simulink model "w3_warplab_trigger_proc"  (Simulink 7.7)
settings: Solver=ode45  StartTime=0.0  StopTime=100  RelTol=1e-3
InitFcn:
  | warplab_trigger_proc_init
StartFcn:
  | warplab_trigger_proc_init
undefined symbols (not defined in the file or in its folder): gcbh, xlBlockLoadCallback, xlGetNormalizedPeriod
libraries: xbsIndex_r4 x817, xbsEDKLib_r4 x1
(part 3 of 6)

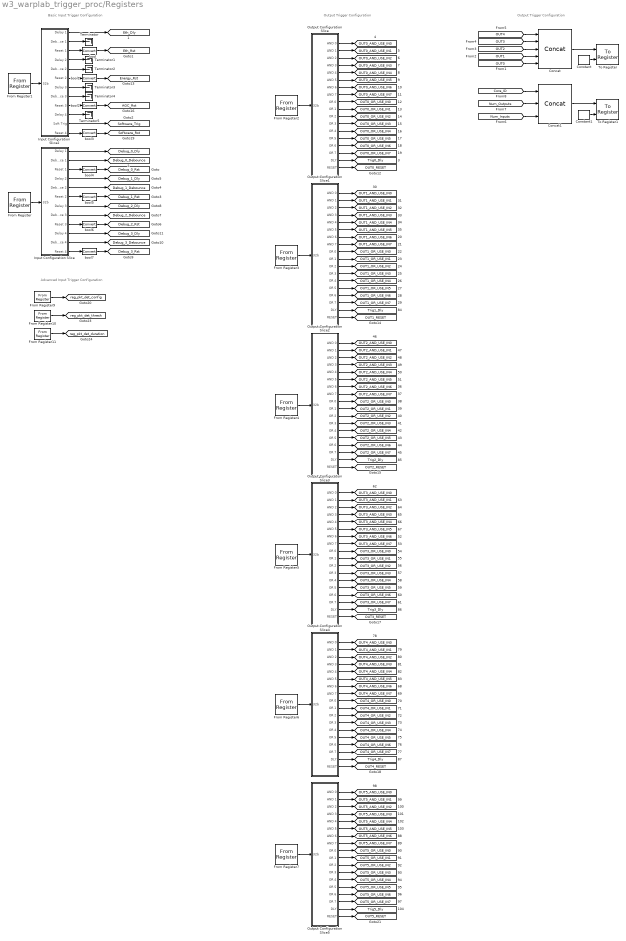
== system w3_warplab_trigger_proc/Registers ==
  note: Basic Input Trigger Configuration
  note: Advanced Input Trigger Configuration
  note: Output Trigger Configuration
  note: Output Trigger Configuration
  Concat : xbsIndex_r4/Concat  num_inputs=5  dbl_ovrd=off  block_type=concat
  Concat1 : xbsIndex_r4/Concat  num_inputs=3  dbl_ovrd=off  block_type=concat
  Constant : xbsIndex_r4/Constant  const=1  gui_display_data_type=Boolean  arith_type=Boolean  n_bits=16  bin_pt=14  preci_type=Single  exp_width=8  frac_width=24  explicit_period=off  period=1  equ=P=C  opselect=C  inp2=PCIN>>17  opr=+  inp1=P  carry=CIN  dbl_ovrd=off  block_type=constant
  Constant1 : xbsIndex_r4/Constant  const=1  gui_display_data_type=Boolean  arith_type=Boolean  n_bits=16  bin_pt=14  preci_type=Single  exp_width=8  frac_width=24  explicit_period=off  period=1  equ=P=C  opselect=C  inp2=PCIN>>17  opr=+  inp1=P  carry=CIN  dbl_ovrd=off  block_type=constant
  From Register : xbsIndex_r4/From Register  shared_memory_name='TRIG_CONF_INBANK1'  init=IN_BANK1  period=1  ownership=Locally owned and initialized  gui_display_data_type=Fixed-point  arith_type=Unsigned  n_bits=32  bin_pt=0  preci_type=Single  dbl_ovrd=off  block_type=fromreg
      settings: AttributesFormatString=<< %<shared_memory_name> >>  infoedit="Register block that reads data to a shared memory register.  Delay of one sample period."
  From Register1 : xbsIndex_r4/From Register  shared_memory_name='TRIG_CONF_INBANK0'  init=IN_BANK0  period=1  ownership=Locally owned and initialized  gui_display_data_type=Fixed-point  arith_type=Unsigned  n_bits=32  bin_pt=0  preci_type=Single  dbl_ovrd=off  block_type=fromreg
      settings: AttributesFormatString=<< %<shared_memory_name> >>  infoedit="Register block that reads data to a shared memory register.  Delay of one sample period."
  From Register10 : xbsIndex_r4/From Register  shared_memory_name='RSSI_PKT_DET_THRESHOLDS'  init=0  period=1  ownership=Locally owned and initialized  gui_display_data_type=Fixed-point  arith_type=Unsigned  n_bits=32  bin_pt=0  preci_type=Single  dbl_ovrd=off  block_type=fromreg
      settings: AttributesFormatString=<< %<shared_memory_name> >>  infoedit="Register block that reads data to a shared memory register.  Delay of one sample period."  block_version=8.2
  From Register11 : xbsIndex_r4/From Register  shared_memory_name='RSSI_PKT_DET_DURATIONS'  init=0  period=1  ownership=Locally owned and initialized  gui_display_data_type=Fixed-point  arith_type=Unsigned  n_bits=32  bin_pt=0  preci_type=Single  dbl_ovrd=off  block_type=fromreg
      settings: AttributesFormatString=<< %<shared_memory_name> >>  infoedit="Register block that reads data to a shared memory register.  Delay of one sample period."  block_version=8.2
  From Register2 : xbsIndex_r4/From Register  shared_memory_name='TRIG_CONF_OUT0'  init=OUT0  period=1  ownership=Locally owned and initialized  gui_display_data_type=Fixed-point  arith_type=Unsigned  n_bits=32  bin_pt=0  preci_type=Single  dbl_ovrd=off  block_type=fromreg
      settings: AttributesFormatString=<< %<shared_memory_name> >>  infoedit="Register block that reads data to a shared memory register.  Delay of one sample period."
  From Register3 : xbsIndex_r4/From Register  shared_memory_name='TRIG_CONF_OUT1'  init=OUT1  period=1  ownership=Locally owned and initialized  gui_display_data_type=Fixed-point  arith_type=Unsigned  n_bits=32  bin_pt=0  preci_type=Single  dbl_ovrd=off  block_type=fromreg
      settings: AttributesFormatString=<< %<shared_memory_name> >>  infoedit="Register block that reads data to a shared memory register.  Delay of one sample period."
  From Register4 : xbsIndex_r4/From Register  shared_memory_name='TRIG_CONF_OUT2'  init=OUT2  period=1  ownership=Locally owned and initialized  gui_display_data_type=Fixed-point  arith_type=Unsigned  n_bits=32  bin_pt=0  preci_type=Single  dbl_ovrd=off  block_type=fromreg
      settings: AttributesFormatString=<< %<shared_memory_name> >>  infoedit="Register block that reads data to a shared memory register.  Delay of one sample period."
  From Register5 : xbsIndex_r4/From Register  shared_memory_name='TRIG_CONF_OUT3'  init=OUT3  period=1  ownership=Locally owned and initialized  gui_display_data_type=Fixed-point  arith_type=Unsigned  n_bits=32  bin_pt=0  preci_type=Single  dbl_ovrd=off  block_type=fromreg
      settings: AttributesFormatString=<< %<shared_memory_name> >>  infoedit="Register block that reads data to a shared memory register.  Delay of one sample period."
  From Register6 : xbsIndex_r4/From Register  shared_memory_name='TRIG_CONF_OUT4'  init=OUT4  period=1  ownership=Locally owned and initialized  gui_display_data_type=Fixed-point  arith_type=Unsigned  n_bits=32  bin_pt=0  preci_type=Single  dbl_ovrd=off  block_type=fromreg
      settings: AttributesFormatString=<< %<shared_memory_name> >>  infoedit="Register block that reads data to a shared memory register.  Delay of one sample period."
  From Register7 : xbsIndex_r4/From Register  shared_memory_name='TRIG_CONF_OUT5'  init=OUT5  period=1  ownership=Locally owned and initialized  gui_display_data_type=Fixed-point  arith_type=Unsigned  n_bits=32  bin_pt=0  preci_type=Single  dbl_ovrd=off  block_type=fromreg
      settings: AttributesFormatString=<< %<shared_memory_name> >>  infoedit="Register block that reads data to a shared memory register.  Delay of one sample period."
  From Register9 : xbsIndex_r4/From Register  shared_memory_name='RSSI_PKT_DET_CONFIG'  init=0  period=1  ownership=Locally owned and initialized  gui_display_data_type=Fixed-point  arith_type=Unsigned  n_bits=32  bin_pt=0  preci_type=Single  dbl_ovrd=off  block_type=fromreg
      settings: AttributesFormatString=<< %<shared_memory_name> >>  infoedit="Register block that reads data to a shared memory register.  Delay of one sample period."  block_version=8.2
  Input Configuration Slice : Subsystem
  Input Configuration Slice2 : Subsystem
  Output Configuration Slice : Subsystem
  Output Configuration Slice1 : Subsystem
  Output Configuration Slice2 : Subsystem
  Output Configuration Slice3 : Subsystem
  Output Configuration Slice4 : Subsystem
  Output Configuration Slice5 : Subsystem
  Terminator{,1..5} (6 alike) : Terminator
  To Register : xbsIndex_r4/To Register  shared_memory_name='TRIG_OUT'  init=0  ownership=Locally owned and initialized  explicit_data_type=on  gui_display_data_type=Fixed-point  arith_type=Unsigned  n_bits=5  bin_pt=0  preci_type=Single  dbl_ovrd=off  block_type=toreg
      settings: AttributesFormatString=<< %<shared_memory_name> >>  infoedit="Register block that writes data to a shared memory register.  Delay of one sample period."
  To Register1 : xbsIndex_r4/To Register  shared_memory_name='CORE_INFO'  init=0  ownership=Locally owned and initialized  explicit_data_type=on  gui_display_data_type=Fixed-point  arith_type=Unsigned  n_bits=24  bin_pt=0  preci_type=Single  dbl_ovrd=off  block_type=toreg
      settings: AttributesFormatString=<< %<shared_memory_name> >>  infoedit="Register block that writes data to a shared memory register.  Delay of one sample period."
  bool{,1..7} (8 alike) : xbsIndex_r4/Convert  gui_display_data_type=Boolean  arith_type=Boolean  n_bits=16  bin_pt=14  float_type=Single  exp_bits=8  fraction_bits=24  quantization=Truncate  overflow=Wrap  en=off  latency=0  dbl_ovrd=off  pipeline=off  block_type=convert
  tag scope: AGC_Rst=global, Debug_0_Debounce=global, Debug_0_Dly=global, Debug_0_Rst=global, Debug_1_Debounce=global, Debug_1_Dly=global, Debug_1_Rst=global, Debug_2_Debounce=global, Debug_2_Dly=global, Debug_2_Rst=global, Debug_3_Debounce=global, Debug_3_Dly=global, Debug_3_Rst=global, Energy_Rst=global, Eth_Dly=global, Eth_Rst=global, OUT0_AND_USE_IN0=global, OUT0_AND_USE_IN1=global, OUT0_AND_USE_IN2=global, OUT0_AND_USE_IN3=global, OUT0_AND_USE_IN4=global, OUT0_AND_USE_IN5=global, OUT0_AND_USE_IN6=global, OUT0_AND_USE_IN7=global, OUT0_OR_USE_IN0=global, OUT0_OR_USE_IN1=global, OUT0_OR_USE_IN2=global, OUT0_OR_USE_IN3=global, OUT0_OR_USE_IN4=global, OUT0_OR_USE_IN5=global, OUT0_OR_USE_IN6=global, OUT0_OR_USE_IN7=global, OUT0_RESET=global, OUT1_AND_USE_IN0=global, OUT1_AND_USE_IN1=global, OUT1_AND_USE_IN2=global, OUT1_AND_USE_IN3=global, OUT1_AND_USE_IN4=global, OUT1_AND_USE_IN5=global, OUT1_AND_USE_IN6=global, OUT1_AND_USE_IN7=global, OUT1_OR_USE_IN0=global, OUT1_OR_USE_IN1=global, OUT1_OR_USE_IN2=global, OUT1_OR_USE_IN3=global, OUT1_OR_USE_IN4=global, OUT1_OR_USE_IN5=global, OUT1_OR_USE_IN6=global, OUT1_OR_USE_IN7=global, OUT1_RESET=global, OUT2_AND_USE_IN0=global, OUT2_AND_USE_IN1=global, OUT2_AND_USE_IN2=global, OUT2_AND_USE_IN3=global, OUT2_AND_USE_IN4=global, OUT2_AND_USE_IN5=global, OUT2_AND_USE_IN6=global, OUT2_AND_USE_IN7=global, OUT2_OR_USE_IN0=global, OUT2_OR_USE_IN1=global, OUT2_OR_USE_IN2=global, OUT2_OR_USE_IN3=global, OUT2_OR_USE_IN4=global, OUT2_OR_USE_IN5=global, OUT2_OR_USE_IN6=global, OUT2_OR_USE_IN7=global, OUT2_RESET=global, OUT3_AND_USE_IN0=global, OUT3_AND_USE_IN1=global, OUT3_AND_USE_IN2=global, OUT3_AND_USE_IN3=global, OUT3_AND_USE_IN4=global, OUT3_AND_USE_IN5=global, OUT3_AND_USE_IN6=global, OUT3_AND_USE_IN7=global, OUT3_OR_USE_IN0=global, OUT3_OR_USE_IN1=global, OUT3_OR_USE_IN2=global, OUT3_OR_USE_IN3=global, OUT3_OR_USE_IN4=global, OUT3_OR_USE_IN5=global, OUT3_OR_USE_IN6=global, OUT3_OR_USE_IN7=global, OUT3_RESET=global, OUT4_AND_USE_IN0=global, OUT4_AND_USE_IN1=global, OUT4_AND_USE_IN2=global, OUT4_AND_USE_IN3=global, OUT4_AND_USE_IN4=global, OUT4_AND_USE_IN5=global, OUT4_AND_USE_IN6=global, OUT4_AND_USE_IN7=global, OUT4_OR_USE_IN0=global, OUT4_OR_USE_IN1=global, OUT4_OR_USE_IN2=global, OUT4_OR_USE_IN3=global, OUT4_OR_USE_IN4=global, OUT4_OR_USE_IN5=global, OUT4_OR_USE_IN6=global, OUT4_OR_USE_IN7=global, OUT4_RESET=global, OUT5_AND_USE_IN0=global, OUT5_AND_USE_IN1=global, OUT5_AND_USE_IN2=global, OUT5_AND_USE_IN3=global, OUT5_AND_USE_IN4=global, OUT5_AND_USE_IN5=global, OUT5_AND_USE_IN6=global, OUT5_AND_USE_IN7=global, OUT5_OR_USE_IN0=global, OUT5_OR_USE_IN1=global, OUT5_OR_USE_IN2=global, OUT5_OR_USE_IN3=global, OUT5_OR_USE_IN4=global, OUT5_OR_USE_IN5=global, OUT5_OR_USE_IN6=global, OUT5_OR_USE_IN7=global, OUT5_RESET=global, Software_Rst=global, Software_Trig=global, Trig0_Dly=global, Trig1_Dly=global, Trig2_Dly=global, Trig3_Dly=global, Trig4_Dly=global, Trig5_Dly=global, reg_pkt_det_config=global, reg_pkt_det_duration=global, reg_pkt_det_thresh=global
  wires:
  Input Configuration Slice/1(Delay 1) -> [Debug_0_Dly]
  Input Configuration Slice/2(Debounce 1) -> [Debug_0_Debounce]
  Input Configuration Slice/3(Reset 1) -> bool4/1
  Input Configuration Slice/4(Delay 2) -> [Debug_1_Dly]
  Input Configuration Slice/5(Debounce 2) -> [Debug_1_Debounce]
  Input Configuration Slice/6(Reset 2) -> bool5/1
  Input Configuration Slice/7(Delay 3) -> [Debug_2_Dly]
  Input Configuration Slice/8(Debounce 3) -> [Debug_2_Debounce]
  Input Configuration Slice/9(Reset 3) -> bool6/1
  Input Configuration Slice/10(Delay 4) -> [Debug_3_Dly]
  Input Configuration Slice/11(Debounce 4) -> [Debug_3_Debounce]
  Input Configuration Slice/12(Reset 4) -> bool7/1
  From Register/1 -> Input Configuration Slice/1(32b)
  Input Configuration Slice2/1(Delay 1) -> [Eth_Dly]
  Input Configuration Slice2/2(Debounce 1) -> Terminator/1
  Input Configuration Slice2/3(Reset 1) -> bool/1
  Input Configuration Slice2/4(Delay 2) -> Terminator1/1
  Input Configuration Slice2/5(Debounce 2) -> Terminator2/1
  Input Configuration Slice2/6(Reset 2) -> bool1/1
  Input Configuration Slice2/7(Delay 3) -> Terminator3/1
  Input Configuration Slice2/8(Debounce 3) -> Terminator4/1
  Input Configuration Slice2/9(Reset 3) -> bool2/1
  Input Configuration Slice2/10(Delay 4) -> Terminator5/1
  Input Configuration Slice2/11(Soft Trig) -> [Software_Trig]
  Input Configuration Slice2/12(Reset 4) -> bool3/1
  From Register1/1 -> Input Configuration Slice2/1(32b)
  From Register9/1 -> [reg_pkt_det_config]
  From Register10/1 -> [reg_pkt_det_thresh]
  From Register11/1 -> [reg_pkt_det_duration]
  From Register2/1 -> Output Configuration Slice/1(32b)
  Output Configuration Slice/1(AND 0) -> [OUT0_AND_USE_IN0]
  Output Configuration Slice/2(AND 1) -> [OUT0_AND_USE_IN1]
  Output Configuration Slice/3(AND 2) -> [OUT0_AND_USE_IN2]
  Output Configuration Slice/4(AND 3) -> [OUT0_AND_USE_IN3]
  Output Configuration Slice/5(AND 4) -> [OUT0_AND_USE_IN4]
  Output Configuration Slice/6(AND 5) -> [OUT0_AND_USE_IN5]
  Output Configuration Slice/7(AND 6) -> [OUT0_AND_USE_IN6]
  Output Configuration Slice/8(AND 7) -> [OUT0_AND_USE_IN7]
  Output Configuration Slice/9(OR 0) -> [OUT0_OR_USE_IN0]
  Output Configuration Slice/10(OR 1) -> [OUT0_OR_USE_IN1]
  Output Configuration Slice/11(OR 2) -> [OUT0_OR_USE_IN2]
  Output Configuration Slice/12(OR 3) -> [OUT0_OR_USE_IN3]
  Output Configuration Slice/13(OR 4) -> [OUT0_OR_USE_IN4]
  Output Configuration Slice/14(OR 5) -> [OUT0_OR_USE_IN5]
  Output Configuration Slice/15(OR 6) -> [OUT0_OR_USE_IN6]
  Output Configuration Slice/16(OR 7) -> [OUT0_OR_USE_IN7]
  Output Configuration Slice/18(RESET) -> [OUT0_RESET]
  Output Configuration Slice1/1(AND 0) -> [OUT1_AND_USE_IN0]
  Output Configuration Slice1/2(AND 1) -> [OUT1_AND_USE_IN1]
  Output Configuration Slice1/3(AND 2) -> [OUT1_AND_USE_IN2]
  Output Configuration Slice1/4(AND 3) -> [OUT1_AND_USE_IN3]
  Output Configuration Slice1/5(AND 4) -> [OUT1_AND_USE_IN4]
  Output Configuration Slice1/6(AND 5) -> [OUT1_AND_USE_IN5]
  Output Configuration Slice1/7(AND 6) -> [OUT1_AND_USE_IN6]
  Output Configuration Slice1/8(AND 7) -> [OUT1_AND_USE_IN7]
  Output Configuration Slice1/9(OR 0) -> [OUT1_OR_USE_IN0]
  Output Configuration Slice1/10(OR 1) -> [OUT1_OR_USE_IN1]
  Output Configuration Slice1/11(OR 2) -> [OUT1_OR_USE_IN2]
  Output Configuration Slice1/12(OR 3) -> [OUT1_OR_USE_IN3]
  Output Configuration Slice1/13(OR 4) -> [OUT1_OR_USE_IN4]
  Output Configuration Slice1/14(OR 5) -> [OUT1_OR_USE_IN5]
  Output Configuration Slice1/15(OR 6) -> [OUT1_OR_USE_IN6]
  Output Configuration Slice1/16(OR 7) -> [OUT1_OR_USE_IN7]
  Output Configuration Slice2/1(AND 0) -> [OUT2_AND_USE_IN0]
  Output Configuration Slice2/2(AND 1) -> [OUT2_AND_USE_IN1]
  Output Configuration Slice2/3(AND 2) -> [OUT2_AND_USE_IN2]
  Output Configuration Slice2/4(AND 3) -> [OUT2_AND_USE_IN3]
  Output Configuration Slice2/5(AND 4) -> [OUT2_AND_USE_IN4]
  Output Configuration Slice2/6(AND 5) -> [OUT2_AND_USE_IN5]
  Output Configuration Slice2/7(AND 6) -> [OUT2_AND_USE_IN6]
  Output Configuration Slice2/8(AND 7) -> [OUT2_AND_USE_IN7]
  Output Configuration Slice2/9(OR 0) -> [OUT2_OR_USE_IN0]
  Output Configuration Slice2/10(OR 1) -> [OUT2_OR_USE_IN1]
  Output Configuration Slice2/11(OR 2) -> [OUT2_OR_USE_IN2]
  Output Configuration Slice2/12(OR 3) -> [OUT2_OR_USE_IN3]
  Output Configuration Slice2/13(OR 4) -> [OUT2_OR_USE_IN4]
  Output Configuration Slice2/14(OR 5) -> [OUT2_OR_USE_IN5]
  Output Configuration Slice2/15(OR 6) -> [OUT2_OR_USE_IN6]
  Output Configuration Slice2/16(OR 7) -> [OUT2_OR_USE_IN7]
  Output Configuration Slice3/1(AND 0) -> [OUT3_AND_USE_IN0]
  Output Configuration Slice3/2(AND 1) -> [OUT3_AND_USE_IN1]
  Output Configuration Slice3/3(AND 2) -> [OUT3_AND_USE_IN2]
  Output Configuration Slice3/4(AND 3) -> [OUT3_AND_USE_IN3]
  Output Configuration Slice3/5(AND 4) -> [OUT3_AND_USE_IN4]
  Output Configuration Slice3/6(AND 5) -> [OUT3_AND_USE_IN5]
  Output Configuration Slice3/7(AND 6) -> [OUT3_AND_USE_IN6]
  Output Configuration Slice3/8(AND 7) -> [OUT3_AND_USE_IN7]
  Output Configuration Slice3/9(OR 0) -> [OUT3_OR_USE_IN0]
  Output Configuration Slice3/10(OR 1) -> [OUT3_OR_USE_IN1]
  Output Configuration Slice3/11(OR 2) -> [OUT3_OR_USE_IN2]
  Output Configuration Slice3/12(OR 3) -> [OUT3_OR_USE_IN3]
  Output Configuration Slice3/13(OR 4) -> [OUT3_OR_USE_IN4]
  Output Configuration Slice3/14(OR 5) -> [OUT3_OR_USE_IN5]
  Output Configuration Slice3/15(OR 6) -> [OUT3_OR_USE_IN6]
  Output Configuration Slice3/16(OR 7) -> [OUT3_OR_USE_IN7]
  Output Configuration Slice4/1(AND 0) -> [OUT4_AND_USE_IN0]
  Output Configuration Slice4/2(AND 1) -> [OUT4_AND_USE_IN1]
  Output Configuration Slice4/3(AND 2) -> [OUT4_AND_USE_IN2]
  Output Configuration Slice4/4(AND 3) -> [OUT4_AND_USE_IN3]
  Output Configuration Slice4/5(AND 4) -> [OUT4_AND_USE_IN4]
  Output Configuration Slice4/6(AND 5) -> [OUT4_AND_USE_IN5]
  Output Configuration Slice4/7(AND 6) -> [OUT4_AND_USE_IN6]
  Output Configuration Slice4/8(AND 7) -> [OUT4_AND_USE_IN7]
  Output Configuration Slice4/9(OR 0) -> [OUT4_OR_USE_IN0]
  Output Configuration Slice4/10(OR 1) -> [OUT4_OR_USE_IN1]
  Output Configuration Slice4/11(OR 2) -> [OUT4_OR_USE_IN2]
  Output Configuration Slice4/12(OR 3) -> [OUT4_OR_USE_IN3]
  Output Configuration Slice4/13(OR 4) -> [OUT4_OR_USE_IN4]
  Output Configuration Slice4/14(OR 5) -> [OUT4_OR_USE_IN5]
  Output Configuration Slice4/15(OR 6) -> [OUT4_OR_USE_IN6]
  Output Configuration Slice4/16(OR 7) -> [OUT4_OR_USE_IN7]
  [OUT4] -> Concat/1
  [OUT3] -> Concat/2
  [OUT2] -> Concat/3
  [OUT1] -> Concat/4
  [OUT0] -> Concat/5
  Concat/1 -> To Register/1
  Constant/1 -> To Register/2
  bool/1 -> [Eth_Rst]
  bool1/1 -> [Energy_Rst]
  bool2/1 -> [AGC_Rst]
  bool3/1 -> [Software_Rst]
  bool4/1 -> [Debug_0_Rst]
  bool5/1 -> [Debug_1_Rst]
  bool6/1 -> [Debug_2_Rst]
  bool7/1 -> [Debug_3_Rst]
  Output Configuration Slice/17(DLY) -> [Trig0_Dly]
  Output Configuration Slice1/17(DLY) -> [Trig1_Dly]
  Output Configuration Slice1/18(RESET) -> [OUT1_RESET]
  Output Configuration Slice2/17(DLY) -> [Trig2_Dly]
  Output Configuration Slice2/18(RESET) -> [OUT2_RESET]
  Output Configuration Slice3/17(DLY) -> [Trig3_Dly]
  Output Configuration Slice3/18(RESET) -> [OUT3_RESET]
  Output Configuration Slice4/17(DLY) -> [Trig4_Dly]
  Output Configuration Slice4/18(RESET) -> [OUT4_RESET]
  From Register3/1 -> Output Configuration Slice1/1(32b)
  From Register4/1 -> Output Configuration Slice2/1(32b)
  From Register5/1 -> Output Configuration Slice3/1(32b)
  From Register6/1 -> Output Configuration Slice4/1(32b)
  Concat1/1 -> To Register1/1
  Constant1/1 -> To Register1/2
  [Core_ID] -> Concat1/1
  [Num_Outputs] -> Concat1/2
  [Num_Inputs] -> Concat1/3
  Output Configuration Slice5/1(AND 0) -> [OUT5_AND_USE_IN0]
  Output Configuration Slice5/2(AND 1) -> [OUT5_AND_USE_IN1]
  Output Configuration Slice5/3(AND 2) -> [OUT5_AND_USE_IN2]
  Output Configuration Slice5/4(AND 3) -> [OUT5_AND_USE_IN3]
  Output Configuration Slice5/5(AND 4) -> [OUT5_AND_USE_IN4]
  Output Configuration Slice5/6(AND 5) -> [OUT5_AND_USE_IN5]
  Output Configuration Slice5/7(AND 6) -> [OUT5_AND_USE_IN6]
  Output Configuration Slice5/8(AND 7) -> [OUT5_AND_USE_IN7]
  Output Configuration Slice5/9(OR 0) -> [OUT5_OR_USE_IN0]
  Output Configuration Slice5/10(OR 1) -> [OUT5_OR_USE_IN1]
  Output Configuration Slice5/11(OR 2) -> [OUT5_OR_USE_IN2]
  Output Configuration Slice5/12(OR 3) -> [OUT5_OR_USE_IN3]
  Output Configuration Slice5/13(OR 4) -> [OUT5_OR_USE_IN4]
  Output Configuration Slice5/14(OR 5) -> [OUT5_OR_USE_IN5]
  Output Configuration Slice5/15(OR 6) -> [OUT5_OR_USE_IN6]
  Output Configuration Slice5/16(OR 7) -> [OUT5_OR_USE_IN7]
  Output Configuration Slice5/17(DLY) -> [Trig5_Dly]
  Output Configuration Slice5/18(RESET) -> [OUT5_RESET]
  From Register7/1 -> Output Configuration Slice5/1(32b)

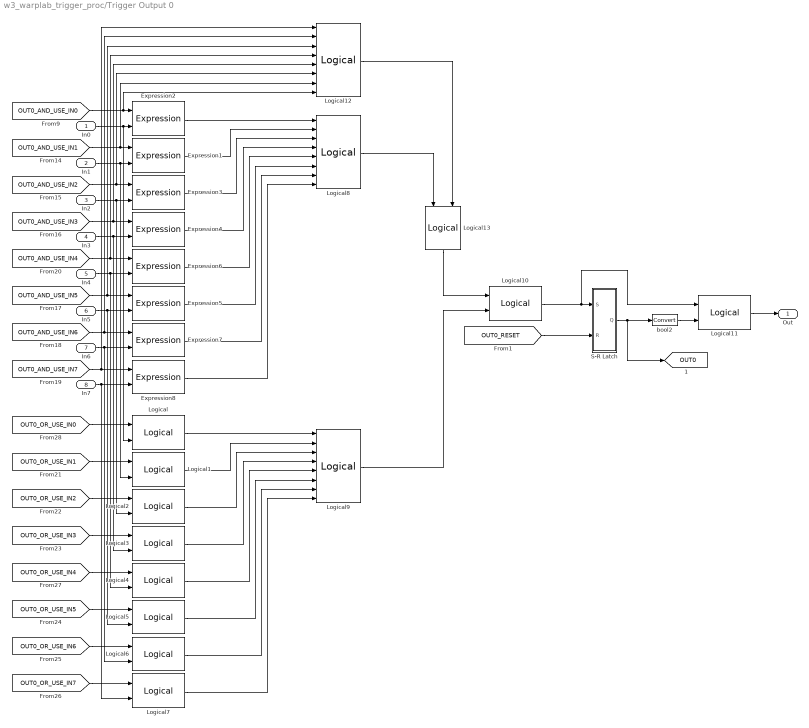
== system w3_warplab_trigger_proc/Trigger Output 0 ==
  In0 : Inport
  In1 : Inport  Port=2
  In2 : Inport  Port=3
  In3 : Inport  Port=4
  In4 : Inport  Port=5
  In5 : Inport  Port=6
  In6 : Inport  Port=7
  In7 : Inport  Port=8
  Expression{1..8} (8 alike) : xbsIndex_r4/Expression  expression=~a | (a & b)  align_bp=on  en=off  latency=0  precision=Full  arith_type=Unsigned  n_bits=16  bin_pt=0  dbl_ovrd=off  block_type=expr
  Logical{,1..7,13} (9 alike) : xbsIndex_r4/Logical  logical_function=AND  inputs=2  en=off  latency=0  precision=Full  arith_type=Unsigned  n_bits=16  bin_pt=0  align_bp=on  dbl_ovrd=off  block_type=logical
  Logical10 : xbsIndex_r4/Logical  logical_function=OR  inputs=2  en=off  latency=0  precision=Full  arith_type=Unsigned  n_bits=16  bin_pt=0  align_bp=on  dbl_ovrd=off  block_type=logical
  Logical11 : xbsIndex_r4/Logical  logical_function=OR  inputs=2  en=off  latency=0  precision=Full  arith_type=Unsigned  n_bits=16  bin_pt=0  align_bp=on  dbl_ovrd=off  block_type=logical
  Logical12 : xbsIndex_r4/Logical  logical_function=OR  inputs=8  en=off  latency=0  precision=Full  arith_type=Unsigned  n_bits=16  bin_pt=0  align_bp=on  dbl_ovrd=off  block_type=logical
  Logical8 : xbsIndex_r4/Logical  logical_function=AND  inputs=8  en=off  latency=0  precision=Full  arith_type=Unsigned  n_bits=16  bin_pt=0  align_bp=on  dbl_ovrd=off  block_type=logical
  Logical9 : xbsIndex_r4/Logical  logical_function=OR  inputs=8  en=off  latency=0  precision=Full  arith_type=Unsigned  n_bits=16  bin_pt=0  align_bp=on  dbl_ovrd=off  block_type=logical
  S-R Latch : Subsystem
  bool2 : xbsIndex_r4/Convert  gui_display_data_type=Boolean  arith_type=Boolean  n_bits=16  bin_pt=14  float_type=Single  exp_bits=8  fraction_bits=24  quantization=Truncate  overflow=Wrap  en=off  latency=0  dbl_ovrd=off  pipeline=off  block_type=convert
  Out : Outport
  tag scope: OUT0=global
  wires:
  [OUT0_AND_USE_IN0] -> Expression2/1, Logical12/8
  [OUT0_AND_USE_IN1] -> Expression1/1, Logical12/7
  [OUT0_AND_USE_IN2] -> Expression3/1, Logical12/6
  [OUT0_AND_USE_IN3] -> Expression4/1, Logical12/5
  [OUT0_AND_USE_IN4] -> Expression6/1, Logical12/4
  [OUT0_AND_USE_IN5] -> Expression5/1, Logical12/3
  [OUT0_AND_USE_IN6] -> Expression7/1, Logical12/2
  [OUT0_AND_USE_IN7] -> Expression8/1, Logical12/1
  In0/1 -> Expression2/2, Logical/2
  In1/1 -> Expression1/2, Logical1/2
  In2/1 -> Expression3/2, Logical2/2
  In3/1 -> Expression4/2, Logical3/2
  In4/1 -> Expression6/2, Logical4/2
  In5/1 -> Expression5/2, Logical5/2
  In6/1 -> Expression7/2, Logical6/2
  In7/1 -> Expression8/2, Logical7/2
  [OUT0_OR_USE_IN0] -> Logical/1
  [OUT0_OR_USE_IN1] -> Logical1/1
  [OUT0_OR_USE_IN2] -> Logical2/1
  [OUT0_OR_USE_IN3] -> Logical3/1
  [OUT0_OR_USE_IN4] -> Logical4/1
  [OUT0_OR_USE_IN5] -> Logical5/1
  [OUT0_OR_USE_IN6] -> Logical6/1
  [OUT0_OR_USE_IN7] -> Logical7/1
  Expression2/1 -> Logical8/1
  Expression1/1 -> Logical8/2
  Expression3/1 -> Logical8/3
  Expression4/1 -> Logical8/4
  Expression6/1 -> Logical8/5
  Expression5/1 -> Logical8/6
  Expression7/1 -> Logical8/7
  Expression8/1 -> Logical8/8
  Logical/1 -> Logical9/1
  Logical1/1 -> Logical9/2
  Logical2/1 -> Logical9/3
  Logical3/1 -> Logical9/4
  Logical4/1 -> Logical9/5
  Logical5/1 -> Logical9/6
  Logical6/1 -> Logical9/7
  Logical7/1 -> Logical9/8
  Logical9/1 -> Logical10/2
  Logical10/1 -> S-R Latch/1(S), Logical11/1
  [OUT0_RESET] -> S-R Latch/2(R)
  S-R Latch/1(Q) -> [OUT0], bool2/1
  Logical11/1 -> Out/1
  bool2/1 -> Logical11/2
  Logical12/1 -> Logical13/2
  Logical13/1 -> Logical10/1
  Logical8/1 -> Logical13/1

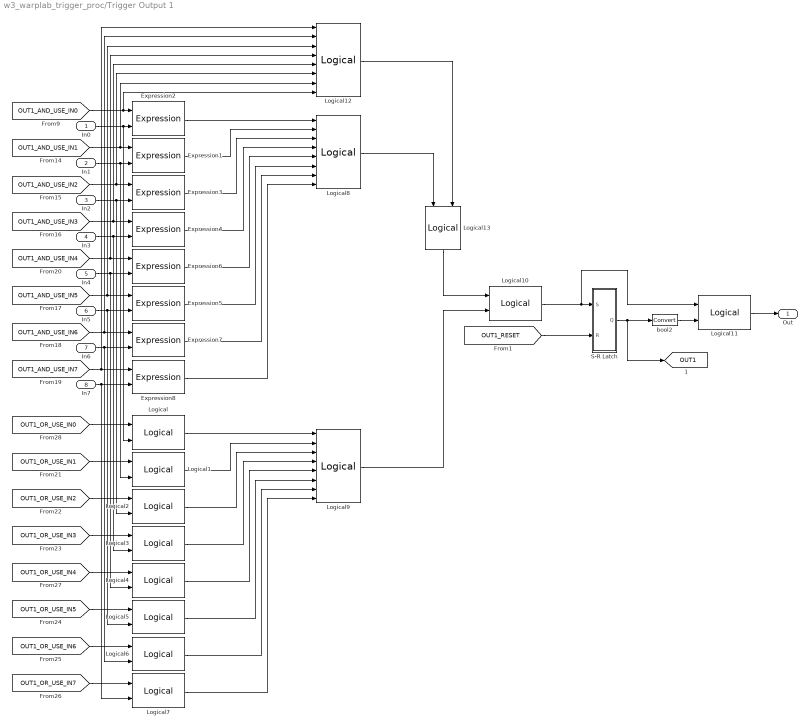
== system w3_warplab_trigger_proc/Trigger Output 1 ==
  In0 : Inport
  In1 : Inport  Port=2
  In2 : Inport  Port=3
  In3 : Inport  Port=4
  In4 : Inport  Port=5
  In5 : Inport  Port=6
  In6 : Inport  Port=7
  In7 : Inport  Port=8
  Expression{1..8} (8 alike) : xbsIndex_r4/Expression  expression=~a | (a & b)  align_bp=on  en=off  latency=0  precision=Full  arith_type=Unsigned  n_bits=16  bin_pt=0  dbl_ovrd=off  block_type=expr
  Logical{,1..7,13} (9 alike) : xbsIndex_r4/Logical  logical_function=AND  inputs=2  en=off  latency=0  precision=Full  arith_type=Unsigned  n_bits=16  bin_pt=0  align_bp=on  dbl_ovrd=off  block_type=logical
  Logical10 : xbsIndex_r4/Logical  logical_function=OR  inputs=2  en=off  latency=0  precision=Full  arith_type=Unsigned  n_bits=16  bin_pt=0  align_bp=on  dbl_ovrd=off  block_type=logical
  Logical11 : xbsIndex_r4/Logical  logical_function=OR  inputs=2  en=off  latency=0  precision=Full  arith_type=Unsigned  n_bits=16  bin_pt=0  align_bp=on  dbl_ovrd=off  block_type=logical
  Logical12 : xbsIndex_r4/Logical  logical_function=OR  inputs=8  en=off  latency=0  precision=Full  arith_type=Unsigned  n_bits=16  bin_pt=0  align_bp=on  dbl_ovrd=off  block_type=logical
  Logical8 : xbsIndex_r4/Logical  logical_function=AND  inputs=8  en=off  latency=0  precision=Full  arith_type=Unsigned  n_bits=16  bin_pt=0  align_bp=on  dbl_ovrd=off  block_type=logical
  Logical9 : xbsIndex_r4/Logical  logical_function=OR  inputs=8  en=off  latency=0  precision=Full  arith_type=Unsigned  n_bits=16  bin_pt=0  align_bp=on  dbl_ovrd=off  block_type=logical
  S-R Latch : Subsystem
  bool2 : xbsIndex_r4/Convert  gui_display_data_type=Boolean  arith_type=Boolean  n_bits=16  bin_pt=14  float_type=Single  exp_bits=8  fraction_bits=24  quantization=Truncate  overflow=Wrap  en=off  latency=0  dbl_ovrd=off  pipeline=off  block_type=convert
  Out : Outport
  tag scope: OUT1=global
  wires:
  Logical8/1 -> Logical13/1
  Logical13/1 -> Logical10/1
  Logical12/1 -> Logical13/2
  bool2/1 -> Logical11/2
  Logical11/1 -> Out/1
  S-R Latch/1(Q) -> bool2/1, [OUT1]
  [OUT1_RESET] -> S-R Latch/2(R)
  Logical10/1 -> Logical11/1, S-R Latch/1(S)
  Logical9/1 -> Logical10/2
  Logical7/1 -> Logical9/8
  Logical6/1 -> Logical9/7
  Logical5/1 -> Logical9/6
  Logical4/1 -> Logical9/5
  Logical3/1 -> Logical9/4
  Logical2/1 -> Logical9/3
  Logical1/1 -> Logical9/2
  Logical/1 -> Logical9/1
  Expression8/1 -> Logical8/8
  Expression7/1 -> Logical8/7
  Expression5/1 -> Logical8/6
  Expression6/1 -> Logical8/5
  Expression4/1 -> Logical8/4
  Expression3/1 -> Logical8/3
  Expression1/1 -> Logical8/2
  Expression2/1 -> Logical8/1
  [OUT1_OR_USE_IN7] -> Logical7/1
  [OUT1_OR_USE_IN6] -> Logical6/1
  [OUT1_OR_USE_IN5] -> Logical5/1
  [OUT1_OR_USE_IN4] -> Logical4/1
  [OUT1_OR_USE_IN3] -> Logical3/1
  [OUT1_OR_USE_IN2] -> Logical2/1
  [OUT1_OR_USE_IN1] -> Logical1/1
  [OUT1_OR_USE_IN0] -> Logical/1
  In7/1 -> Logical7/2, Expression8/2
  In6/1 -> Logical6/2, Expression7/2
  In5/1 -> Logical5/2, Expression5/2
  In4/1 -> Logical4/2, Expression6/2
  In3/1 -> Logical3/2, Expression4/2
  In2/1 -> Logical2/2, Expression3/2
  In1/1 -> Logical1/2, Expression1/2
  In0/1 -> Logical/2, Expression2/2
  [OUT1_AND_USE_IN7] -> Logical12/1, Expression8/1
  [OUT1_AND_USE_IN6] -> Logical12/2, Expression7/1
  [OUT1_AND_USE_IN5] -> Logical12/3, Expression5/1
  [OUT1_AND_USE_IN4] -> Logical12/4, Expression6/1
  [OUT1_AND_USE_IN3] -> Logical12/5, Expression4/1
  [OUT1_AND_USE_IN2] -> Logical12/6, Expression3/1
  [OUT1_AND_USE_IN1] -> Logical12/7, Expression1/1
  [OUT1_AND_USE_IN0] -> Logical12/8, Expression2/1

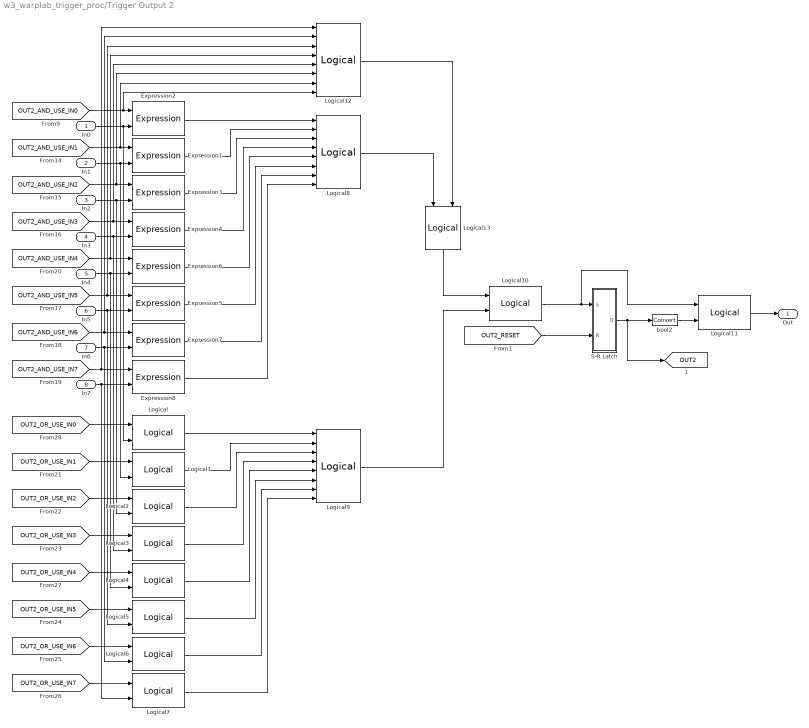
== system w3_warplab_trigger_proc/Trigger Output 2 ==
  In0 : Inport
  In1 : Inport  Port=2
  In2 : Inport  Port=3
  In3 : Inport  Port=4
  In4 : Inport  Port=5
  In5 : Inport  Port=6
  In6 : Inport  Port=7
  In7 : Inport  Port=8
  Expression{1..8} (8 alike) : xbsIndex_r4/Expression  expression=~a | (a & b)  align_bp=on  en=off  latency=0  precision=Full  arith_type=Unsigned  n_bits=16  bin_pt=0  dbl_ovrd=off  block_type=expr
  Logical{,1..7,13} (9 alike) : xbsIndex_r4/Logical  logical_function=AND  inputs=2  en=off  latency=0  precision=Full  arith_type=Unsigned  n_bits=16  bin_pt=0  align_bp=on  dbl_ovrd=off  block_type=logical
  Logical10 : xbsIndex_r4/Logical  logical_function=OR  inputs=2  en=off  latency=0  precision=Full  arith_type=Unsigned  n_bits=16  bin_pt=0  align_bp=on  dbl_ovrd=off  block_type=logical
  Logical11 : xbsIndex_r4/Logical  logical_function=OR  inputs=2  en=off  latency=0  precision=Full  arith_type=Unsigned  n_bits=16  bin_pt=0  align_bp=on  dbl_ovrd=off  block_type=logical
  Logical12 : xbsIndex_r4/Logical  logical_function=OR  inputs=8  en=off  latency=0  precision=Full  arith_type=Unsigned  n_bits=16  bin_pt=0  align_bp=on  dbl_ovrd=off  block_type=logical
  Logical8 : xbsIndex_r4/Logical  logical_function=AND  inputs=8  en=off  latency=0  precision=Full  arith_type=Unsigned  n_bits=16  bin_pt=0  align_bp=on  dbl_ovrd=off  block_type=logical
  Logical9 : xbsIndex_r4/Logical  logical_function=OR  inputs=8  en=off  latency=0  precision=Full  arith_type=Unsigned  n_bits=16  bin_pt=0  align_bp=on  dbl_ovrd=off  block_type=logical
  S-R Latch : Subsystem
  bool2 : xbsIndex_r4/Convert  gui_display_data_type=Boolean  arith_type=Boolean  n_bits=16  bin_pt=14  float_type=Single  exp_bits=8  fraction_bits=24  quantization=Truncate  overflow=Wrap  en=off  latency=0  dbl_ovrd=off  pipeline=off  block_type=convert
  Out : Outport
  tag scope: OUT2=global
  wires:
  [OUT2_AND_USE_IN0] -> Expression2/1, Logical12/8
  [OUT2_AND_USE_IN1] -> Expression1/1, Logical12/7
  [OUT2_AND_USE_IN2] -> Expression3/1, Logical12/6
  [OUT2_AND_USE_IN3] -> Expression4/1, Logical12/5
  [OUT2_AND_USE_IN4] -> Expression6/1, Logical12/4
  [OUT2_AND_USE_IN5] -> Expression5/1, Logical12/3
  [OUT2_AND_USE_IN6] -> Expression7/1, Logical12/2
  [OUT2_AND_USE_IN7] -> Expression8/1, Logical12/1
  In0/1 -> Expression2/2, Logical/2
  In1/1 -> Expression1/2, Logical1/2
  In2/1 -> Expression3/2, Logical2/2
  In3/1 -> Expression4/2, Logical3/2
  In4/1 -> Expression6/2, Logical4/2
  In5/1 -> Expression5/2, Logical5/2
  In6/1 -> Expression7/2, Logical6/2
  In7/1 -> Expression8/2, Logical7/2
  [OUT2_OR_USE_IN0] -> Logical/1
  [OUT2_OR_USE_IN1] -> Logical1/1
  [OUT2_OR_USE_IN2] -> Logical2/1
  [OUT2_OR_USE_IN3] -> Logical3/1
  [OUT2_OR_USE_IN4] -> Logical4/1
  [OUT2_OR_USE_IN5] -> Logical5/1
  [OUT2_OR_USE_IN6] -> Logical6/1
  [OUT2_OR_USE_IN7] -> Logical7/1
  Expression2/1 -> Logical8/1
  Expression1/1 -> Logical8/2
  Expression3/1 -> Logical8/3
  Expression4/1 -> Logical8/4
  Expression6/1 -> Logical8/5
  Expression5/1 -> Logical8/6
  Expression7/1 -> Logical8/7
  Expression8/1 -> Logical8/8
  Logical/1 -> Logical9/1
  Logical1/1 -> Logical9/2
  Logical2/1 -> Logical9/3
  Logical3/1 -> Logical9/4
  Logical4/1 -> Logical9/5
  Logical5/1 -> Logical9/6
  Logical6/1 -> Logical9/7
  Logical7/1 -> Logical9/8
  Logical9/1 -> Logical10/2
  Logical10/1 -> S-R Latch/1(S), Logical11/1
  [OUT2_RESET] -> S-R Latch/2(R)
  S-R Latch/1(Q) -> [OUT2], bool2/1
  Logical11/1 -> Out/1
  bool2/1 -> Logical11/2
  Logical12/1 -> Logical13/2
  Logical13/1 -> Logical10/1
  Logical8/1 -> Logical13/1

== system w3_warplab_trigger_proc/Trigger Output 3 ==
  In0 : Inport
  In1 : Inport  Port=2
  In2 : Inport  Port=3
  In3 : Inport  Port=4
  In4 : Inport  Port=5
  In5 : Inport  Port=6
  In6 : Inport  Port=7
  In7 : Inport  Port=8
  Expression{1..8} (8 alike) : xbsIndex_r4/Expression  expression=~a | (a & b)  align_bp=on  en=off  latency=0  precision=Full  arith_type=Unsigned  n_bits=16  bin_pt=0  dbl_ovrd=off  block_type=expr
  Logical{,1..7,13} (9 alike) : xbsIndex_r4/Logical  logical_function=AND  inputs=2  en=off  latency=0  precision=Full  arith_type=Unsigned  n_bits=16  bin_pt=0  align_bp=on  dbl_ovrd=off  block_type=logical
  Logical10 : xbsIndex_r4/Logical  logical_function=OR  inputs=2  en=off  latency=0  precision=Full  arith_type=Unsigned  n_bits=16  bin_pt=0  align_bp=on  dbl_ovrd=off  block_type=logical
  Logical11 : xbsIndex_r4/Logical  logical_function=OR  inputs=2  en=off  latency=0  precision=Full  arith_type=Unsigned  n_bits=16  bin_pt=0  align_bp=on  dbl_ovrd=off  block_type=logical
  Logical12 : xbsIndex_r4/Logical  logical_function=OR  inputs=8  en=off  latency=0  precision=Full  arith_type=Unsigned  n_bits=16  bin_pt=0  align_bp=on  dbl_ovrd=off  block_type=logical
  Logical8 : xbsIndex_r4/Logical  logical_function=AND  inputs=8  en=off  latency=0  precision=Full  arith_type=Unsigned  n_bits=16  bin_pt=0  align_bp=on  dbl_ovrd=off  block_type=logical
  Logical9 : xbsIndex_r4/Logical  logical_function=OR  inputs=8  en=off  latency=0  precision=Full  arith_type=Unsigned  n_bits=16  bin_pt=0  align_bp=on  dbl_ovrd=off  block_type=logical
  S-R Latch : Subsystem
  bool2 : xbsIndex_r4/Convert  gui_display_data_type=Boolean  arith_type=Boolean  n_bits=16  bin_pt=14  float_type=Single  exp_bits=8  fraction_bits=24  quantization=Truncate  overflow=Wrap  en=off  latency=0  dbl_ovrd=off  pipeline=off  block_type=convert
  Out : Outport
  tag scope: OUT3=global
  wires:
  Logical8/1 -> Logical13/1
  Logical13/1 -> Logical10/1
  Logical12/1 -> Logical13/2
  bool2/1 -> Logical11/2
  Logical11/1 -> Out/1
  S-R Latch/1(Q) -> bool2/1, [OUT3]
  [OUT3_RESET] -> S-R Latch/2(R)
  Logical10/1 -> Logical11/1, S-R Latch/1(S)
  Logical9/1 -> Logical10/2
  Logical7/1 -> Logical9/8
  Logical6/1 -> Logical9/7
  Logical5/1 -> Logical9/6
  Logical4/1 -> Logical9/5
  Logical3/1 -> Logical9/4
  Logical2/1 -> Logical9/3
  Logical1/1 -> Logical9/2
  Logical/1 -> Logical9/1
  Expression8/1 -> Logical8/8
  Expression7/1 -> Logical8/7
  Expression5/1 -> Logical8/6
  Expression6/1 -> Logical8/5
  Expression4/1 -> Logical8/4
  Expression3/1 -> Logical8/3
  Expression1/1 -> Logical8/2
  Expression2/1 -> Logical8/1
  [OUT3_OR_USE_IN7] -> Logical7/1
  [OUT3_OR_USE_IN6] -> Logical6/1
  [OUT3_OR_USE_IN5] -> Logical5/1
  [OUT3_OR_USE_IN4] -> Logical4/1
  [OUT3_OR_USE_IN3] -> Logical3/1
  [OUT3_OR_USE_IN2] -> Logical2/1
  [OUT3_OR_USE_IN1] -> Logical1/1
  [OUT3_OR_USE_IN0] -> Logical/1
  In7/1 -> Logical7/2, Expression8/2
  In6/1 -> Logical6/2, Expression7/2
  In5/1 -> Logical5/2, Expression5/2
  In4/1 -> Logical4/2, Expression6/2
  In3/1 -> Logical3/2, Expression4/2
  In2/1 -> Logical2/2, Expression3/2
  In1/1 -> Logical1/2, Expression1/2
  In0/1 -> Logical/2, Expression2/2
  [OUT3_OR_USE_IN7] -> Logical12/1, Expression8/1
  [OUT3_OR_USE_IN6] -> Logical12/2, Expression7/1
  [OUT3_OR_USE_IN5] -> Logical12/3, Expression5/1
  [OUT3_OR_USE_IN4] -> Logical12/4, Expression6/1
  [OUT3_OR_USE_IN3] -> Logical12/5, Expression4/1
  [OUT3_OR_USE_IN2] -> Logical12/6, Expression3/1
  [OUT3_OR_USE_IN1] -> Logical12/7, Expression1/1
  [OUT3_OR_USE_IN0] -> Logical12/8, Expression2/1

== system w3_warplab_trigger_proc/Trigger Output 4 ==
  In0 : Inport
  In1 : Inport  Port=2
  In2 : Inport  Port=3
  In3 : Inport  Port=4
  In4 : Inport  Port=5
  In5 : Inport  Port=6
  In6 : Inport  Port=7
  In7 : Inport  Port=8
  Expression{1..8} (8 alike) : xbsIndex_r4/Expression  expression=~a | (a & b)  align_bp=on  en=off  latency=0  precision=Full  arith_type=Unsigned  n_bits=16  bin_pt=0  dbl_ovrd=off  block_type=expr
  Logical{,1..7,13} (9 alike) : xbsIndex_r4/Logical  logical_function=AND  inputs=2  en=off  latency=0  precision=Full  arith_type=Unsigned  n_bits=16  bin_pt=0  align_bp=on  dbl_ovrd=off  block_type=logical
  Logical10 : xbsIndex_r4/Logical  logical_function=OR  inputs=2  en=off  latency=0  precision=Full  arith_type=Unsigned  n_bits=16  bin_pt=0  align_bp=on  dbl_ovrd=off  block_type=logical
  Logical11 : xbsIndex_r4/Logical  logical_function=OR  inputs=2  en=off  latency=0  precision=Full  arith_type=Unsigned  n_bits=16  bin_pt=0  align_bp=on  dbl_ovrd=off  block_type=logical
  Logical12 : xbsIndex_r4/Logical  logical_function=OR  inputs=8  en=off  latency=0  precision=Full  arith_type=Unsigned  n_bits=16  bin_pt=0  align_bp=on  dbl_ovrd=off  block_type=logical
  Logical8 : xbsIndex_r4/Logical  logical_function=AND  inputs=8  en=off  latency=0  precision=Full  arith_type=Unsigned  n_bits=16  bin_pt=0  align_bp=on  dbl_ovrd=off  block_type=logical
  Logical9 : xbsIndex_r4/Logical  logical_function=OR  inputs=8  en=off  latency=0  precision=Full  arith_type=Unsigned  n_bits=16  bin_pt=0  align_bp=on  dbl_ovrd=off  block_type=logical
  S-R Latch : Subsystem
  bool2 : xbsIndex_r4/Convert  gui_display_data_type=Boolean  arith_type=Boolean  n_bits=16  bin_pt=14  float_type=Single  exp_bits=8  fraction_bits=24  quantization=Truncate  overflow=Wrap  en=off  latency=0  dbl_ovrd=off  pipeline=off  block_type=convert
  Out : Outport
  tag scope: OUT4=global
  wires:
  [OUT4_OR_USE_IN0] -> Expression2/1, Logical12/8
  [OUT4_OR_USE_IN1] -> Expression1/1, Logical12/7
  [OUT4_OR_USE_IN2] -> Expression3/1, Logical12/6
  [OUT4_OR_USE_IN3] -> Expression4/1, Logical12/5
  [OUT4_OR_USE_IN4] -> Expression6/1, Logical12/4
  [OUT4_OR_USE_IN5] -> Expression5/1, Logical12/3
  [OUT4_OR_USE_IN6] -> Expression7/1, Logical12/2
  [OUT4_OR_USE_IN7] -> Expression8/1, Logical12/1
  In0/1 -> Expression2/2, Logical/2
  In1/1 -> Expression1/2, Logical1/2
  In2/1 -> Expression3/2, Logical2/2
  In3/1 -> Expression4/2, Logical3/2
  In4/1 -> Expression6/2, Logical4/2
  In5/1 -> Expression5/2, Logical5/2
  In6/1 -> Expression7/2, Logical6/2
  In7/1 -> Expression8/2, Logical7/2
  [OUT4_OR_USE_IN0] -> Logical/1
  [OUT4_OR_USE_IN1] -> Logical1/1
  [OUT4_OR_USE_IN2] -> Logical2/1
  [OUT4_OR_USE_IN3] -> Logical3/1
  [OUT4_OR_USE_IN4] -> Logical4/1
  [OUT4_OR_USE_IN5] -> Logical5/1
  [OUT4_OR_USE_IN6] -> Logical6/1
  [OUT4_OR_USE_IN7] -> Logical7/1
  Expression2/1 -> Logical8/1
  Expression1/1 -> Logical8/2
  Expression3/1 -> Logical8/3
  Expression4/1 -> Logical8/4
  Expression6/1 -> Logical8/5
  Expression5/1 -> Logical8/6
  Expression7/1 -> Logical8/7
  Expression8/1 -> Logical8/8
  Logical/1 -> Logical9/1
  Logical1/1 -> Logical9/2
  Logical2/1 -> Logical9/3
  Logical3/1 -> Logical9/4
  Logical4/1 -> Logical9/5
  Logical5/1 -> Logical9/6
  Logical6/1 -> Logical9/7
  Logical7/1 -> Logical9/8
  Logical9/1 -> Logical10/2
  Logical10/1 -> S-R Latch/1(S), Logical11/1
  [OUT4_RESET] -> S-R Latch/2(R)
  S-R Latch/1(Q) -> [OUT4], bool2/1
  Logical11/1 -> Out/1
  bool2/1 -> Logical11/2
  Logical12/1 -> Logical13/2
  Logical13/1 -> Logical10/1
  Logical8/1 -> Logical13/1

== system w3_warplab_trigger_proc/Trigger Output 5 ==
  In0 : Inport
  In1 : Inport  Port=2
  In2 : Inport  Port=3
  In3 : Inport  Port=4
  In4 : Inport  Port=5
  In5 : Inport  Port=6
  In6 : Inport  Port=7
  In7 : Inport  Port=8
  Expression{1..8} (8 alike) : xbsIndex_r4/Expression  expression=~a | (a & b)  align_bp=on  en=off  latency=0  precision=Full  arith_type=Unsigned  n_bits=16  bin_pt=0  dbl_ovrd=off  block_type=expr
  Logical{,1..7,13} (9 alike) : xbsIndex_r4/Logical  logical_function=AND  inputs=2  en=off  latency=0  precision=Full  arith_type=Unsigned  n_bits=16  bin_pt=0  align_bp=on  dbl_ovrd=off  block_type=logical
  Logical10 : xbsIndex_r4/Logical  logical_function=OR  inputs=2  en=off  latency=0  precision=Full  arith_type=Unsigned  n_bits=16  bin_pt=0  align_bp=on  dbl_ovrd=off  block_type=logical
  Logical11 : xbsIndex_r4/Logical  logical_function=OR  inputs=2  en=off  latency=0  precision=Full  arith_type=Unsigned  n_bits=16  bin_pt=0  align_bp=on  dbl_ovrd=off  block_type=logical
  Logical12 : xbsIndex_r4/Logical  logical_function=OR  inputs=8  en=off  latency=0  precision=Full  arith_type=Unsigned  n_bits=16  bin_pt=0  align_bp=on  dbl_ovrd=off  block_type=logical
  Logical8 : xbsIndex_r4/Logical  logical_function=AND  inputs=8  en=off  latency=0  precision=Full  arith_type=Unsigned  n_bits=16  bin_pt=0  align_bp=on  dbl_ovrd=off  block_type=logical
  Logical9 : xbsIndex_r4/Logical  logical_function=OR  inputs=8  en=off  latency=0  precision=Full  arith_type=Unsigned  n_bits=16  bin_pt=0  align_bp=on  dbl_ovrd=off  block_type=logical
  S-R Latch : Subsystem
  bool2 : xbsIndex_r4/Convert  gui_display_data_type=Boolean  arith_type=Boolean  n_bits=16  bin_pt=14  float_type=Single  exp_bits=8  fraction_bits=24  quantization=Truncate  overflow=Wrap  en=off  latency=0  dbl_ovrd=off  pipeline=off  block_type=convert
  Out : Outport
  tag scope: OUT5=global
  wires:
  Logical8/1 -> Logical13/1
  Logical13/1 -> Logical10/1
  Logical12/1 -> Logical13/2
  bool2/1 -> Logical11/2
  Logical11/1 -> Out/1
  S-R Latch/1(Q) -> bool2/1, [OUT5]
  [OUT5_RESET] -> S-R Latch/2(R)
  Logical10/1 -> Logical11/1, S-R Latch/1(S)
  Logical9/1 -> Logical10/2
  Logical7/1 -> Logical9/8
  Logical6/1 -> Logical9/7
  Logical5/1 -> Logical9/6
  Logical4/1 -> Logical9/5
  Logical3/1 -> Logical9/4
  Logical2/1 -> Logical9/3
  Logical1/1 -> Logical9/2
  Logical/1 -> Logical9/1
  Expression8/1 -> Logical8/8
  Expression7/1 -> Logical8/7
  Expression5/1 -> Logical8/6
  Expression6/1 -> Logical8/5
  Expression4/1 -> Logical8/4
  Expression3/1 -> Logical8/3
  Expression1/1 -> Logical8/2
  Expression2/1 -> Logical8/1
  [OUT5_OR_USE_IN7] -> Logical7/1
  [OUT5_OR_USE_IN6] -> Logical6/1
  [OUT5_OR_USE_IN5] -> Logical5/1
  [OUT5_OR_USE_IN4] -> Logical4/1
  [OUT5_OR_USE_IN3] -> Logical3/1
  [OUT5_OR_USE_IN2] -> Logical2/1
  [OUT5_OR_USE_IN1] -> Logical1/1
  [OUT5_OR_USE_IN0] -> Logical/1
  In7/1 -> Logical7/2, Expression8/2
  In6/1 -> Logical6/2, Expression7/2
  In5/1 -> Logical5/2, Expression5/2
  In4/1 -> Logical4/2, Expression6/2
  In3/1 -> Logical3/2, Expression4/2
  In2/1 -> Logical2/2, Expression3/2
  In1/1 -> Logical1/2, Expression1/2
  In0/1 -> Logical/2, Expression2/2
  [OUT5_OR_USE_IN7] -> Logical12/1, Expression8/1
  [OUT5_OR_USE_IN6] -> Logical12/2, Expression7/1
  [OUT5_OR_USE_IN5] -> Logical12/3, Expression5/1
  [OUT5_OR_USE_IN4] -> Logical12/4, Expression6/1
  [OUT5_OR_USE_IN3] -> Logical12/5, Expression4/1
  [OUT5_OR_USE_IN2] -> Logical12/6, Expression3/1
  [OUT5_OR_USE_IN1] -> Logical12/7, Expression1/1
  [OUT5_OR_USE_IN0] -> Logical12/8, Expression2/1

== system w3_warplab_trigger_proc/Trigger Sources ==
  AGC : Subsystem
  Addressable Shift Register{,3..6} (5 alike) : xbsIndex_r4/Addressable Shift Register  infer_latency=off  depth=32  initVector=[0]  en=off  dbl_ovrd=off  use_behavioral_HDL=off  Optimization=Resource  block_type=addrsr
      settings: infoedit="Delay of configurable length.  Any element in the delay line can be addressed and driven onto the output port.<br><br>Hardware notes: This block is implemented using SRL16s. If Virtex-4 or Spartan-3 device is used, multiple SRLC16s are cascaded together."
  Debug 0 : Subsystem
  Debug 1 : Subsystem
  Debug 2 : Subsystem
  Debug 3 : Subsystem
  Energy : Subsystem
  Ethernet : Subsystem
  Register{,1..7} (8 alike) : xbsIndex_r4/Register  init=0  rst=on  en=off  dbl_ovrd=off  block_type=register
  Software : Subsystem
  bool{1..7,10} (8 alike) : xbsIndex_r4/Convert  gui_display_data_type=Boolean  arith_type=Boolean  n_bits=16  bin_pt=14  float_type=Single  exp_bits=8  fraction_bits=24  quantization=Truncate  overflow=Wrap  en=off  latency=0  dbl_ovrd=off  pipeline=off  block_type=convert
  Out0 : Outport
  Out1 : Outport  Port=2
  Out2 : Outport  Port=3
  Out3 : Outport  Port=4
  Out4 : Outport  Port=5
  Out5 : Outport  Port=6
  Out6 : Outport  Port=7
  Out7 : Outport  Port=8
  wires:
  Ethernet/1(Trigger) -> Register/1
  [Eth_Rst] -> Register/2
  Energy/1(Trigger) -> Register1/1
  [Energy_Rst] -> Register1/2
  AGC/1(Trigger) -> Register2/1
  [AGC_Rst] -> Register2/2
  Debug 0/1(Trigger) -> Register3/1
  [Debug_0_Rst] -> Register3/2
  Debug 1/1(Trigger) -> Register4/1
  [Debug_1_Rst] -> Register4/2
  Debug 2/1(Trigger) -> Register5/1
  [Debug_2_Rst] -> Register5/2
  Debug 3/1(Trigger) -> Register6/1
  [Debug_3_Rst] -> Register6/2
  Register/1 -> Addressable Shift Register/1
  [Eth_Dly] -> Addressable Shift Register/2
  [Debug_0_Dly] -> Addressable Shift Register3/2
  Register3/1 -> Addressable Shift Register3/1
  [Debug_1_Dly] -> Addressable Shift Register4/2
  Register4/1 -> Addressable Shift Register4/1
  [Debug_2_Dly] -> Addressable Shift Register5/2
  Register5/1 -> Addressable Shift Register5/1
  [Debug_3_Dly] -> Addressable Shift Register6/2
  Register6/1 -> Addressable Shift Register6/1
  Software/1(Trigger) -> Register7/1
  [Software_Rst] -> Register7/2
  Addressable Shift Register/1 -> bool10/1
  Register1/1 -> bool1/1
  Register2/1 -> bool2/1
  Register7/1 -> bool3/1
  Addressable Shift Register3/1 -> bool4/1
  Addressable Shift Register4/1 -> bool5/1
  Addressable Shift Register5/1 -> bool6/1
  Addressable Shift Register6/1 -> bool7/1
  bool10/1 -> Out0/1
  bool1/1 -> Out1/1
  bool2/1 -> Out2/1
  bool3/1 -> Out3/1
  bool4/1 -> Out4/1
  bool5/1 -> Out5/1
  bool6/1 -> Out6/1
  bool7/1 -> Out7/1

== system w3_warplab_trigger_proc/Registers/Input Configuration Slice ==
  32b : Inport
  (LSB+0):(LSB+4) : xbsIndex_r4/Slice  nbits=5  boolean_output=off  mode=Lower Bit Location + Width  bit1=0  base1=MSB of Input  bit0=0  base0=LSB of Input  dbl_ovrd=off  block_type=slice
  (LSB+16):(LSB+20) : xbsIndex_r4/Slice  nbits=5  boolean_output=off  mode=Lower Bit Location + Width  bit1=0  base1=MSB of Input  bit0=16  base0=LSB of Input  dbl_ovrd=off  block_type=slice
  (LSB+24):(LSB+28) : xbsIndex_r4/Slice  nbits=5  boolean_output=off  mode=Lower Bit Location + Width  bit1=0  base1=MSB of Input  bit0=24  base0=LSB of Input  dbl_ovrd=off  block_type=slice
  (LSB+8):(LSB+12) : xbsIndex_r4/Slice  nbits=5  boolean_output=off  mode=Lower Bit Location + Width  bit1=0  base1=MSB of Input  bit0=8  base0=LSB of Input  dbl_ovrd=off  block_type=slice
  LSB+13 : xbsIndex_r4/Slice  nbits=1  boolean_output=off  mode=Lower Bit Location + Width  bit1=0  base1=MSB of Input  bit0=13  base0=LSB of Input  dbl_ovrd=off  block_type=slice
  LSB+14 : xbsIndex_r4/Slice  nbits=1  boolean_output=off  mode=Lower Bit Location + Width  bit1=0  base1=MSB of Input  bit0=14  base0=LSB of Input  dbl_ovrd=off  block_type=slice
  LSB+21 : xbsIndex_r4/Slice  nbits=1  boolean_output=off  mode=Lower Bit Location + Width  bit1=0  base1=MSB of Input  bit0=21  base0=LSB of Input  dbl_ovrd=off  block_type=slice
  LSB+22 : xbsIndex_r4/Slice  nbits=1  boolean_output=off  mode=Lower Bit Location + Width  bit1=0  base1=MSB of Input  bit0=22  base0=LSB of Input  dbl_ovrd=off  block_type=slice
  LSB+29 : xbsIndex_r4/Slice  nbits=1  boolean_output=off  mode=Lower Bit Location + Width  bit1=0  base1=MSB of Input  bit0=29  base0=LSB of Input  dbl_ovrd=off  block_type=slice
  LSB+31 : xbsIndex_r4/Slice  nbits=1  boolean_output=off  mode=Lower Bit Location + Width  bit1=0  base1=MSB of Input  bit0=31  base0=LSB of Input  dbl_ovrd=off  block_type=slice
  LSB+5 : xbsIndex_r4/Slice  nbits=1  boolean_output=off  mode=Lower Bit Location + Width  bit1=0  base1=MSB of Input  bit0=5  base0=LSB of Input  dbl_ovrd=off  block_type=slice
  LSB+6 : xbsIndex_r4/Slice  nbits=1  boolean_output=off  mode=Lower Bit Location + Width  bit1=0  base1=MSB of Input  bit0=6  base0=LSB of Input  dbl_ovrd=off  block_type=slice
  Delay 1 : Outport
  Debounce 1 : Outport  Port=2
  Reset 1 : Outport  Port=3
  Delay 2 : Outport  Port=4
  Debounce 2 : Outport  Port=5
  Reset 2 : Outport  Port=6
  Delay 3 : Outport  Port=7
  Debounce 3 : Outport  Port=8
  Reset 3 : Outport  Port=9
  Delay 4 : Outport  Port=10
  Debounce 4 : Outport  Port=11
  Reset 4 : Outport  Port=12
  wires:
  32b/1 -> LSB+31/1, LSB+29/1, (LSB+24):(LSB+28)/1, LSB+22/1, LSB+21/1, (LSB+16):(LSB+20)/1, LSB+14/1, LSB+13/1, (LSB+8):(LSB+12)/1, LSB+6/1, LSB+5/1, (LSB+0):(LSB+4)/1
  (LSB+0):(LSB+4)/1 -> Delay 1/1
  LSB+5/1 -> Debounce 1/1
  LSB+6/1 -> Reset 1/1
  (LSB+8):(LSB+12)/1 -> Delay 2/1
  LSB+13/1 -> Debounce 2/1
  LSB+14/1 -> Reset 2/1
  (LSB+16):(LSB+20)/1 -> Delay 3/1
  LSB+21/1 -> Debounce 3/1
  LSB+22/1 -> Reset 3/1
  (LSB+24):(LSB+28)/1 -> Delay 4/1
  LSB+29/1 -> Debounce 4/1
  LSB+31/1 -> Reset 4/1
